simulink library "TimeSpoolingController_ul"  (R2018b)
settings: Solver=VariableStepAuto  StartTime=0.0  StopTime=10.0  RelTol=1e-3
undefined symbols (not defined in the file or in its folder): pathCtrl, runSpoolSpeed
settings Model: Creator=James Reed  LastModifiedBy=jldanie5

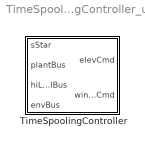
== system TimeSpoolingController_ul ==
  TimeSpoolingController : Subsystem

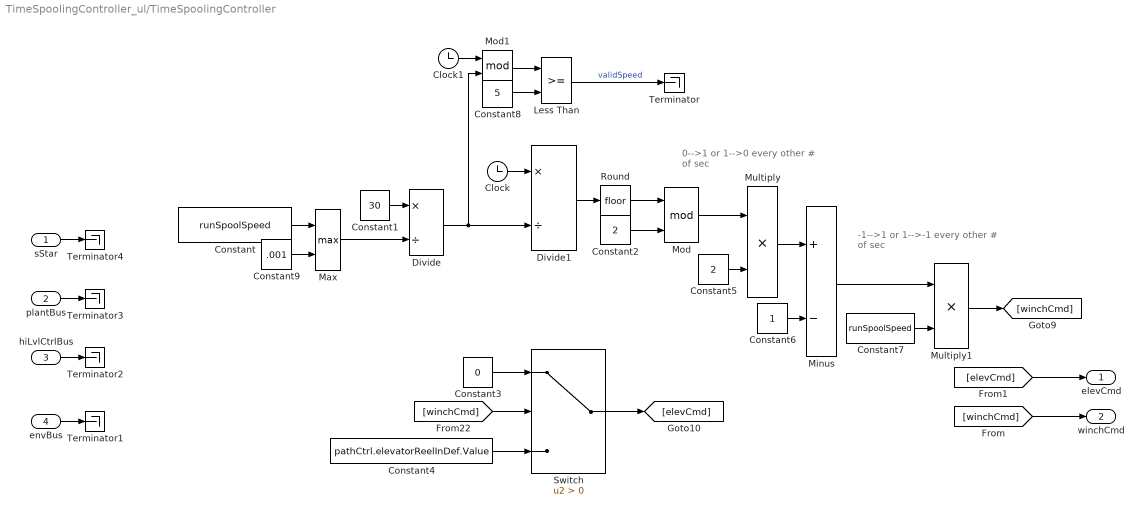
== system TimeSpoolingController_ul/TimeSpoolingController ==
  note: 0-->1 or 1-->0
      | every other # of sec
  note: -1-->1 or 1-->-1
      | every other # of sec
  "sStar " : Inport
  plantBus : Inport  Port=2  OutDataTypeStr=Bus: plantBus
  hiLvlCtrlBus : Inport  Port=3  OutDataTypeStr=Bus: hiLvlCtrlBus
  envBus : Inport  Port=4  OutDataTypeStr=Bus: envBus
  Clock : Clock
  Clock1 : Clock
  Constant : Constant  Value=runSpoolSpeed
  Constant1 : Constant  Value=30
  Constant2 : Constant  Value=2
  Constant3 : Constant  Value=0
  Constant4 : Constant  Value=pathCtrl.elevatorReelInDef.Value
  Constant5 : Constant  Value=2
  Constant6 : Constant
  Constant7 : Constant  Value=runSpoolSpeed
  Constant8 : Constant  Value=5
  Constant9 : Constant  Value=.001
  Divide : Product  Inputs=*/
  Divide1 : Product  Inputs=*/
  Less Than : RelationalOperator  OutDataTypeStr=boolean  RndMeth=Simplest
  Max : MinMax  Function=max  Inputs=2
  Minus : Sum  Inputs=+-
  Mod : Math  Operator=mod  SaturateOnIntegerOverflow=on
  Mod1 : Math  Operator=mod  SaturateOnIntegerOverflow=on
  Multiply : Product
  Multiply1 : Product
  Round : Rounding
  Switch : Switch  Criteria=u2 > Threshold
  Terminator{,1..4} (5 alike) : Terminator
  elevCmd : Outport
  "winchCmd " : Outport  Port=2
  wires:
  [winchCmd] -> "winchCmd "/1
  hiLvlCtrlBus/1 -> Terminator2/1
  [elevCmd] -> elevCmd/1
  envBus/1 -> Terminator1/1
  Switch/1 -> [elevCmd]
  Constant4/1 -> Switch/3
  Constant3/1 -> Switch/1
  [winchCmd] -> Switch/2
  plantBus/1 -> Terminator3/1
  "sStar "/1 -> Terminator4/1
  Constant1/1 -> Divide/1
  Clock/1 -> Divide1/1
  Divide/1 -> Divide1/2, Mod1/2
  Divide1/1 -> Round/1
  Round/1 -> Mod/1
  Constant2/1 -> Mod/2
  Mod/1 -> Multiply/1
  Constant5/1 -> Multiply/2
  Multiply/1 -> Minus/1
  Constant6/1 -> Minus/2
  Minus/1 -> Multiply1/1
  Constant7/1 -> Multiply1/2
  Multiply1/1 -> [winchCmd]
  Clock1/1 -> Mod1/1
  Mod1/1 -> Less Than/1
  Constant8/1 -> Less Than/2
  Less Than/1 -> Terminator/1  "validSpeed"
  Constant/1 -> Max/1
  Max/1 -> Divide/2
  Constant9/1 -> Max/2
